simulink model "gm_sampleModel1590_sub"  (R2023a)
settings: Solver=VariableStepAuto  StartTime=0.0  StopTime=10.0  RelTol=1e-3
libraries: simulink x1, hdlsllib x1
settings Model: Creator=user1  LastModifiedBy=user1
settings OptimizationCC: BlockReduction=off  ConditionallyExecuteInputs=off
settings DebuggingCC: InheritedTsInSrcMsg=none

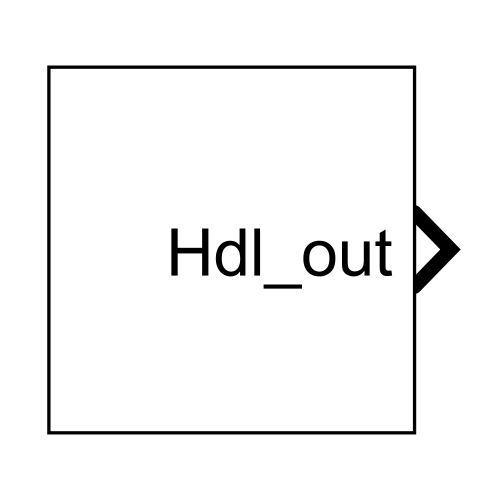
[thumbnail: Simulink's stored preview of the top-level diagram]
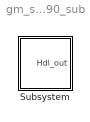
== system gm_sampleModel1590_sub ==
  Subsystem : Subsystem

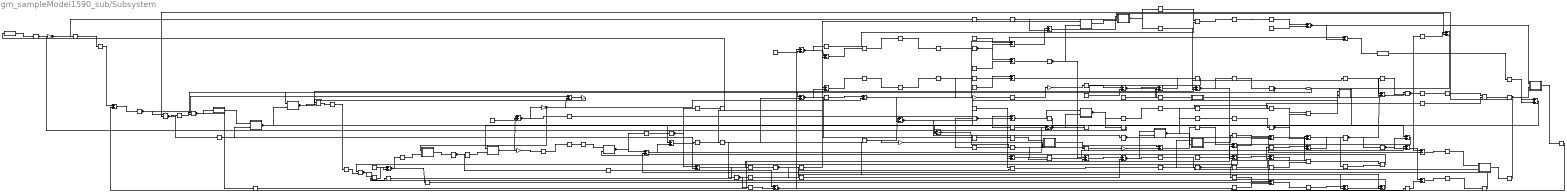
== system gm_sampleModel1590_sub/Subsystem ==
  Reshape{,1..6} (7 alike) : Reshape
  cfblk1 : Subsystem  mask(Detect Fall Nonpositive){vinit=double(0), InputProcessing=Elements as channels (sample based), OutDataTypeStr=uint8}
      mask prompts: vinit "Simulink:masks:InitialCondition_MP"; InputProcessing "Simulink:masks:InputProcessing_MP"; OutDataTypeStr "Simulink:masks:OutputDataType_MP"
      mask help: Simulink:masks:DetectFallNonpositive_MD
      mask init:
      | InputProcessing = 'Elements as channels (sample based)';
      | OutDataTypeStr = 'uint8';
      | vinit = double(0);
      mask TypeOptions InputProcessing: Simulink:masks:ColumnsAsChannelsFrameBased | Simulink:masks:ElementsAsChannelsSampleBased
      mask TypeOptions OutDataTypeStr: Simulink:masks:uint8 | Simulink:masks:boolean
      mask Display: fprintf('U <= 0\n&  NOT\nU/z <= 0')
  cfblk{10..11,18,20,23,31,51,76,82,92..93,104,106,117,120,125,127,131,137,139,145} (21 alike) : Signum  SampleTime=1
  cfblk{43,50,54,72,95,100,114,142} (8 alike) : Gain  Gain="fi(0,0,8,7,\"hex\",\"80\")"  ParamDataTypeStr=fixdt(0, 8, 7)  OutDataTypeStr=uint8  SampleTime=1
  cfblk{27,38,70..71,101,123,130,133,136,150} (10 alike) : Sum  Inputs=+  OutDataTypeStr=uint8
  cfblk102_inst : Subsystem
  cfblk{19,42,58,61,63,77,87,103,110,112,115,140} (12 alike) : Product  Inputs=*/  OutDataTypeStr=uint8  RndMeth=Zero  SaturateOnIntegerOverflow=on  SampleTime=1
  cfblk{4,33,45,60,74,84,89,105,121..122,134,147} (12 alike) : Sum  AccumDataTypeStr=uint8  OutDataTypeStr=uint8  RndMeth=Nearest  SampleTime=1
  cfblk105_const_val : Constant  Value=0  VectorParams1D=off  OutDataTypeStr=uint8  SampleTime=1
  cfblk{8,29,34,36,48..49,56..57,64,66,78,85..86,94,97,107,111,129,143..144} (20 alike) : Sum  AccumDataTypeStr=uint8  OutDataTypeStr=uint8  SampleTime=1
  cfblk{16,21,24,28,30,55,62,68,81,96,109,118} (12 alike) : Abs  SampleTime=1  OutDataTypeStr=uint8  SaturateOnIntegerOverflow=off
  cfblk{6,25..26,35,37,39..40,47,52..53,69,80,91,99,113,116,141,152} (18 alike) : MinMax  OutDataTypeStr=uint8
  cfblk{5,15,59,67,73,79,83,90,119,124,128,132} (12 alike) : Sum  Inputs=+-  AccumDataTypeStr=uint8  OutDataTypeStr=uint8  SampleTime=1
  cfblk121_const_val : Constant  Value=0  VectorParams1D=off  OutDataTypeStr=uint8  SampleTime=1
  cfblk122_const_val : Constant  Value=0  VectorParams1D=off  OutDataTypeStr=uint8  SampleTime=1
  cfblk126_inst : Subsystem
  cfblk134_const_val : Constant  Value=0  VectorParams1D=off  OutDataTypeStr=uint8  SampleTime=1
  cfblk135_inst : Subsystem
  cfblk13_inst : Subsystem
  cfblk146_inst : Subsystem
  cfblk147_const_val : Constant  Value=0  VectorParams1D=off  OutDataTypeStr=uint8  SampleTime=1
  cfblk148_inst : Subsystem
  cfblk149_inst : Subsystem
  cfblk158 : Constant  OutDataTypeStr=uint8  SampleTime=1
  cfblk159 : Constant  OutDataTypeStr=uint8  SampleTime=1
  cfblk160 : Constant  Value=0  VectorParams1D=off  OutDataTypeStr=uint8  SampleTime=1
  cfblk161 : Subsystem
  cfblk162 : Subsystem
  cfblk164 : Switch  Threshold=double(0)  OutDataTypeStr=uint8  SampleTime=1  SaturateOnIntegerOverflow=off  InputSameDT=off
  cfblk165 : Switch  Threshold=double(0)  OutDataTypeStr=uint8  SampleTime=1  SaturateOnIntegerOverflow=off  InputSameDT=off
  cfblk{166..190} (25 alike) : Delay  DelayLength=double(2)  InitialCondition=0  SampleTime=1
  cfblk17_inst : Subsystem
  cfblk{191..192,194..195} (4 alike) : DataTypeConversion  OutDataTypeStr=fixdt(0,8,0)
  cfblk193 : DataTypeConversion  OutDataTypeStr=uint8  SampleTime=1  SaturateOnIntegerOverflow=off  RndMeth=Floor
  cfblk2 : simulink/Logic and Bit Operations/Detect Increase  vinit=0.0  OutDataTypeStr=uint8
      settings: LibrarySourceBlock=|
      | hdlsllib/Logic and Bit
      | Operations/Detect
      | Increase
  cfblk3 : hdlsllib/Logic and Bit Operations/Bit Concat  numInputs=2
  cfblk32_inst : Subsystem
  cfblk33_const_val : Constant  Value=0  VectorParams1D=off  OutDataTypeStr=uint8  SampleTime=1
  cfblk44_inst : Subsystem
  cfblk45_const_val : Constant  Value=0  VectorParams1D=off  OutDataTypeStr=uint8  SampleTime=1
  cfblk4_const_val : Constant  Value=0  VectorParams1D=off  OutDataTypeStr=uint8  SampleTime=1
  cfblk60_const_val : Constant  Value=0  VectorParams1D=off  OutDataTypeStr=uint8  SampleTime=1
  cfblk65_inst : Subsystem
  cfblk74_const_val : Constant  Value=0  VectorParams1D=off  OutDataTypeStr=uint8  SampleTime=1
  cfblk84_const_val : Constant  Value=0  VectorParams1D=off  OutDataTypeStr=uint8  SampleTime=1
  cfblk88_inst : Subsystem
  cfblk89_const_val : Constant  Value=0  VectorParams1D=off  OutDataTypeStr=uint8  SampleTime=1
  cfblk98_inst : Subsystem
  cfblk9_inst : Subsystem
  Hdl_out : Outport  OutDataTypeStr=uint8  SampleTime=1
  wires:
  cfblk1/1(Y) -> cfblk191/1
  cfblk10/1 -> Reshape3/1
  cfblk100/1 -> cfblk97/2
  cfblk101/1 -> cfblk70/1
  cfblk102_inst/1(out1) -> cfblk176/1, cfblk80/1
  cfblk103/1 -> cfblk120/1, cfblk162/1(In1)
  cfblk104/1 -> cfblk146_inst/2(in2)
  cfblk105/1 -> cfblk63/1
  cfblk106/1 -> cfblk188/1
  cfblk107/1 -> cfblk48/2, cfblk20/1, cfblk145/1, cfblk13_inst/1(in1)
  Reshape/1 -> cfblk122/1
  cfblk109/1 -> cfblk126_inst/1(in1), cfblk119/2
  cfblk11/1 -> cfblk82/1
  cfblk110/1 -> cfblk123/1
  cfblk111/1 -> cfblk124/2, cfblk26/1
  cfblk112/1 -> cfblk84/1
  cfblk113/1 -> cfblk98_inst/1(in1)
  cfblk114/1 -> cfblk141/1
  cfblk115/1 -> cfblk146_inst/1(in1)
  cfblk116/1 -> cfblk57/2, cfblk115/2
  cfblk117/1 -> cfblk29/1, cfblk189/1
  cfblk118/1 -> cfblk90/2, cfblk137/1, cfblk107/2
  cfblk119/1 -> cfblk113/1
  Reshape1/1 -> cfblk194/1
  cfblk120/1 -> cfblk124/1
  cfblk121/1 -> cfblk185/1
  cfblk122/1 -> cfblk49/2
  cfblk123/1 -> cfblk98_inst/2(in2), cfblk149_inst/1(in1)
  cfblk124/1 -> cfblk105/1
  cfblk125/1 -> cfblk177/1
  cfblk126_inst/1(out1) -> cfblk149_inst/2(in2), cfblk10/1, cfblk186/1
  cfblk127/1 -> cfblk4/1
  cfblk128/1 -> cfblk16/1
  cfblk129/1 -> cfblk6/1
  cfblk13_inst/1(out1) -> cfblk65_inst/2(in2)
  cfblk130/1 -> cfblk101/1
  cfblk131/1 -> cfblk94/1
  cfblk132/1 -> cfblk2/1
  cfblk133/1 -> cfblk8/2, cfblk5/2
  cfblk134/1 -> cfblk104/1, cfblk54/1
  cfblk135_inst/1(out1) -> cfblk111/1, cfblk61/2
  cfblk136/1 -> cfblk106/1
  cfblk137/1 -> cfblk24/1, cfblk174/1
  cfblk139/1 -> cfblk8/1
  Reshape2/1 -> cfblk79/1
  cfblk140/1 -> cfblk139/1, Reshape1/1, cfblk119/1
  cfblk141/1 -> cfblk95/1
  cfblk142/1 -> cfblk136/1
  cfblk143/1 -> cfblk39/1
  cfblk144/1 -> cfblk77/1
  cfblk145/1 -> cfblk66/1
  cfblk146_inst/1(out1) -> cfblk129/1
  cfblk147/1 -> cfblk40/1
  cfblk148_inst/1(out1) -> cfblk85/2, cfblk135_inst/2(in2)
  cfblk149_inst/1(out1) -> cfblk172/1
  cfblk15/1 -> cfblk5/1
  cfblk150/1 -> cfblk56/2, cfblk144/2
  Reshape3/1 -> cfblk116/1
  cfblk152/1 -> cfblk167/1
  cfblk158/1 -> cfblk59/1, cfblk72/1
  cfblk159/1 -> cfblk15/1
  cfblk16/1 -> cfblk93/1
  cfblk160/1 -> cfblk63/2
  cfblk161/1(Out1) -> cfblk184/1
  cfblk162/1(Out1) -> cfblk148_inst/1(in1)
  cfblk164/1 -> cfblk18/1, cfblk102_inst/2(in2)
  cfblk165/1 -> cfblk81/1, cfblk38/1, cfblk52/1
  cfblk166/1 -> cfblk32_inst/2(in2)
  cfblk167/1 -> cfblk73/2
  cfblk168/1 -> cfblk79/2
  cfblk169/1 -> cfblk36/1
  cfblk17_inst/1(out1) -> cfblk92/1
  cfblk170/1 -> cfblk111/2
  cfblk171/1 -> cfblk58/2
  cfblk172/1 -> cfblk49/1
  cfblk173/1 -> cfblk19/2
  cfblk174/1 -> cfblk94/2
  cfblk175/1 -> cfblk17_inst/2(in2)
  cfblk176/1 -> cfblk164/1
  cfblk177/1 -> cfblk115/1
  cfblk178/1 -> cfblk165/2
  cfblk179/1 -> cfblk164/3
  cfblk18/1 -> cfblk165/1
  cfblk180/1 -> cfblk9_inst/1(in1)
  cfblk181/1 -> cfblk34/2
  cfblk182/1 -> cfblk128/2
  cfblk183/1 -> cfblk67/1
  cfblk184/1 -> cfblk140/2
  cfblk185/1 -> cfblk135_inst/1(in1)
  cfblk186/1 -> cfblk195/1
  cfblk187/1 -> cfblk143/1
  cfblk188/1 -> cfblk44_inst/1(in1)
  cfblk189/1 -> cfblk192/1
  cfblk19/1 -> Reshape4/1, cfblk47/1
  cfblk190/1 -> cfblk103/2, Hdl_out/1
  cfblk191/1 -> cfblk109/1, cfblk50/1
  cfblk192/1 -> cfblk1/1(U)
  cfblk193/1 -> cfblk88_inst/2(in2), cfblk36/2
  cfblk194/1 -> cfblk3/1
  cfblk195/1 -> cfblk3/2
  cfblk2/1 -> cfblk169/1
  cfblk20/1 -> cfblk164/2, cfblk42/1
  cfblk21/1 -> cfblk53/1
  cfblk23/1 -> cfblk21/1
  cfblk24/1 -> cfblk110/2
  cfblk25/1 -> cfblk78/1, cfblk19/1
  cfblk26/1 -> cfblk190/1
  cfblk27/1 -> cfblk83/2
  cfblk28/1 -> cfblk100/1
  cfblk29/1 -> cfblk86/2
  cfblk3/1 -> cfblk193/1
  cfblk30/1 -> cfblk56/1
  cfblk31/1 -> cfblk77/2
  cfblk32_inst/1(out1) -> cfblk134/1, cfblk142/1
  cfblk33/1 -> Reshape5/1
  cfblk34/1 -> cfblk55/1, cfblk126_inst/2(in2)
  cfblk35/1 -> cfblk87/1
  cfblk36/1 -> cfblk32_inst/1(in1)
  cfblk37/1 -> Reshape2/1
  cfblk38/1 -> cfblk85/1, cfblk45/1, cfblk179/1
  cfblk39/1 -> cfblk67/2, cfblk150/1
  cfblk4/1 -> cfblk62/1, cfblk121/1
  cfblk40/1 -> cfblk64/1
  Reshape4/1 -> cfblk103/1
  cfblk42/1 -> cfblk57/1
  cfblk43/1 -> cfblk61/1
  cfblk44_inst/1(out1) -> cfblk73/1, cfblk91/1
  cfblk45/1 -> cfblk102_inst/1(in1), cfblk178/1
  Reshape5/1 -> cfblk86/1, cfblk13_inst/2(in2)
  cfblk47/1 -> cfblk29/2, cfblk148_inst/2(in2)
  cfblk48/1 -> cfblk130/1
  cfblk49/1 -> cfblk143/2
  cfblk5/1 -> cfblk65_inst/1(in1)
  cfblk50/1 -> cfblk37/1, cfblk71/1
  cfblk51/1 -> cfblk76/1, cfblk187/1
  cfblk52/1 -> cfblk110/1
  cfblk53/1 -> cfblk64/2, cfblk182/1, cfblk181/1
  cfblk54/1 -> cfblk78/2, cfblk66/2, cfblk17_inst/1(in1)
  cfblk55/1 -> cfblk51/1
  cfblk56/1 -> cfblk83/1
  cfblk57/1 -> cfblk171/1
  cfblk58/1 -> cfblk44_inst/2(in2)
  cfblk59/1 -> cfblk165/3, cfblk144/1
  cfblk6/1 -> cfblk48/1, cfblk118/1
  cfblk60/1 -> cfblk88_inst/1(in1), cfblk132/2
  cfblk61/1 -> cfblk68/1
  cfblk62/1 -> cfblk161/1(In1)
  cfblk63/1 -> cfblk58/1
  cfblk64/1 -> cfblk90/1
  cfblk65_inst/1(out1) -> cfblk170/1, cfblk35/1
  cfblk66/1 -> cfblk59/2, cfblk132/1
  cfblk67/1 -> cfblk140/1
  cfblk68/1 -> cfblk31/1
  cfblk69/1 -> cfblk33/1, cfblk15/2
  cfblk70/1 -> Reshape6/1, cfblk114/1
  cfblk71/1 -> cfblk133/1
  cfblk72/1 -> cfblk97/1
  cfblk73/1 -> cfblk9_inst/2(in2), cfblk129/2
  cfblk74/1 -> cfblk183/1
  Reshape6/1 -> cfblk74/1
  cfblk76/1 -> cfblk147/1
  cfblk77/1 -> cfblk23/1, cfblk112/1
  cfblk78/1 -> cfblk43/1
  cfblk79/1 -> cfblk25/1
  cfblk8/1 -> cfblk107/1
  cfblk80/1 -> cfblk125/1
  cfblk81/1 -> cfblk180/1
  cfblk82/1 -> cfblk60/1
  cfblk83/1 -> cfblk152/1
  cfblk84/1 -> cfblk30/1, cfblk175/1
  cfblk85/1 -> cfblk42/2
  cfblk86/1 -> cfblk34/1
  cfblk87/1 -> cfblk11/1
  cfblk88_inst/1(out1) -> cfblk168/1
  cfblk89/1 -> cfblk128/1, cfblk99/1
  cfblk9_inst/1(out1) -> cfblk28/1
  cfblk90/1 -> cfblk112/2
  cfblk91/1 -> cfblk117/1
  cfblk92/1 -> cfblk131/1, cfblk166/1
  cfblk93/1 -> cfblk96/1
  cfblk94/1 -> cfblk89/1, cfblk27/1
  cfblk95/1 -> cfblk127/1
  cfblk96/1 -> cfblk69/1
  cfblk97/1 -> Reshape/1
  cfblk98_inst/1(out1) -> cfblk173/1
  cfblk99/1 -> cfblk87/2
  cfblk105_const_val/1 -> cfblk105/2
  cfblk121_const_val/1 -> cfblk121/2
  cfblk122_const_val/1 -> cfblk122/2
  cfblk134_const_val/1 -> cfblk134/2
  cfblk147_const_val/1 -> cfblk147/2
  cfblk33_const_val/1 -> cfblk33/2
  cfblk4_const_val/1 -> cfblk4/2
  cfblk45_const_val/1 -> cfblk45/2
  cfblk60_const_val/1 -> cfblk60/2
  cfblk74_const_val/1 -> cfblk74/2
  cfblk84_const_val/1 -> cfblk84/2
  cfblk89_const_val/1 -> cfblk89/2

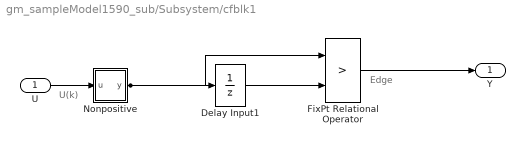
== system gm_sampleModel1590_sub/Subsystem/cfblk1 ==
  note: U(k)
  note: Edge
  U : Inport  OutDataTypeStr=uint8  SampleTime=1
  Delay Input1 : UnitDelay  Description=Store in Global RAM  DisableCoverage=on  InitialCondition=vinit  SampleTime=-1  HasFrameUpgradeWarning=on
  FixPt Relational Operator : RelationalOperator  Operator=>  OutDataTypeStr=fixdt(0, 8)  ZeroCross=off  InputSameDT=off
  Nonpositive : Subsystem  mask(Compare To Zero){relop=<=, OutDataTypeStr=boolean, ZeroCross=off}
      mask prompts: relop "Simulink:masks:Operator_MP"; OutDataTypeStr "Simulink:masks:OutputDataType_MP"; ZeroCross "Simulink:masks:EnableZerocrossingDetection_MP"
      mask help: Simulink:masks:CompareToZero_MD
      mask init:
      | OutDataTypeStr = 'boolean';
      | ZeroCross = 'off';
      | blkName = 'sampleModel1590_sub/Subsystem/cfblk1/Nonpositive';
      | relop = '<=';
      | setValue = 'boolean';
      mask TypeOptions relop: == | ~= | < | <= | >= | >
      mask TypeOptions OutDataTypeStr: Simulink:masks:uint8 | Simulink:masks:boolean
      mask Callback ZeroCross: sl('zeroCrossEnable', gcbh);
      mask Display: disp([relop,' 0'])
  Y : Outport  SampleTime=1
  wires:
  U/1 -> Nonpositive/1(u)
  Delay Input1/1 -> FixPt Relational Operator/2
  FixPt Relational Operator/1 -> Y/1
  Nonpositive/1(y) -> FixPt Relational Operator/1, Delay Input1/1

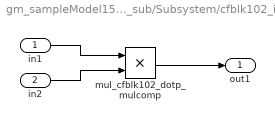
== system gm_sampleModel1590_sub/Subsystem/cfblk102_inst ==
  in1 : Inport  OutDataTypeStr=uint8  SampleTime=1
  in2 : Inport  Port=2  OutDataTypeStr=uint8  SampleTime=1
  mul_cfblk102_dotp_mulcomp : Product  Inputs=**  OutDataTypeStr=uint8  SampleTime=1
  out1 : Outport  OutDataTypeStr=uint8  SampleTime=1
  wires:
  in1/1 -> mul_cfblk102_dotp_mulcomp/1
  in2/1 -> mul_cfblk102_dotp_mulcomp/2
  mul_cfblk102_dotp_mulcomp/1 -> out1/1

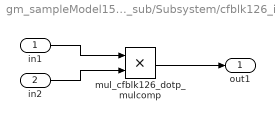
== system gm_sampleModel1590_sub/Subsystem/cfblk126_inst ==
  in1 : Inport  OutDataTypeStr=uint8  SampleTime=1
  in2 : Inport  Port=2  OutDataTypeStr=uint8  SampleTime=1
  mul_cfblk126_dotp_mulcomp : Product  Inputs=**  OutDataTypeStr=uint8  SampleTime=1
  out1 : Outport  OutDataTypeStr=uint8  SampleTime=1
  wires:
  in1/1 -> mul_cfblk126_dotp_mulcomp/1
  in2/1 -> mul_cfblk126_dotp_mulcomp/2
  mul_cfblk126_dotp_mulcomp/1 -> out1/1

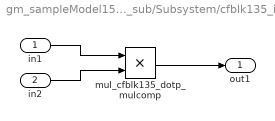
== system gm_sampleModel1590_sub/Subsystem/cfblk135_inst ==
  in1 : Inport  OutDataTypeStr=uint8  SampleTime=1
  in2 : Inport  Port=2  OutDataTypeStr=uint8  SampleTime=1
  mul_cfblk135_dotp_mulcomp : Product  Inputs=**  OutDataTypeStr=uint8  SampleTime=1
  out1 : Outport  OutDataTypeStr=uint8  SampleTime=1
  wires:
  in1/1 -> mul_cfblk135_dotp_mulcomp/1
  in2/1 -> mul_cfblk135_dotp_mulcomp/2
  mul_cfblk135_dotp_mulcomp/1 -> out1/1

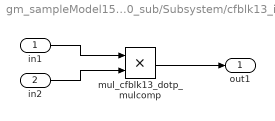
== system gm_sampleModel1590_sub/Subsystem/cfblk13_inst ==
  in1 : Inport  OutDataTypeStr=uint8  SampleTime=1
  in2 : Inport  Port=2  OutDataTypeStr=uint8  SampleTime=1
  mul_cfblk13_dotp_mulcomp : Product  Inputs=**  OutDataTypeStr=uint8  SampleTime=1
  out1 : Outport  OutDataTypeStr=uint8  SampleTime=1
  wires:
  in1/1 -> mul_cfblk13_dotp_mulcomp/1
  in2/1 -> mul_cfblk13_dotp_mulcomp/2
  mul_cfblk13_dotp_mulcomp/1 -> out1/1

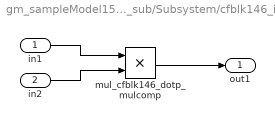
== system gm_sampleModel1590_sub/Subsystem/cfblk146_inst ==
  in1 : Inport  OutDataTypeStr=uint8  SampleTime=1
  in2 : Inport  Port=2  OutDataTypeStr=uint8  SampleTime=1
  mul_cfblk146_dotp_mulcomp : Product  Inputs=**  OutDataTypeStr=uint8  SampleTime=1
  out1 : Outport  OutDataTypeStr=uint8  SampleTime=1
  wires:
  in1/1 -> mul_cfblk146_dotp_mulcomp/1
  in2/1 -> mul_cfblk146_dotp_mulcomp/2
  mul_cfblk146_dotp_mulcomp/1 -> out1/1

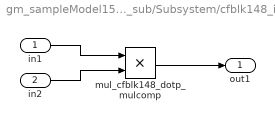
== system gm_sampleModel1590_sub/Subsystem/cfblk148_inst ==
  in1 : Inport  OutDataTypeStr=uint8  SampleTime=1
  in2 : Inport  Port=2  OutDataTypeStr=uint8  SampleTime=1
  mul_cfblk148_dotp_mulcomp : Product  Inputs=**  OutDataTypeStr=uint8  SampleTime=1
  out1 : Outport  OutDataTypeStr=uint8  SampleTime=1
  wires:
  in1/1 -> mul_cfblk148_dotp_mulcomp/1
  in2/1 -> mul_cfblk148_dotp_mulcomp/2
  mul_cfblk148_dotp_mulcomp/1 -> out1/1

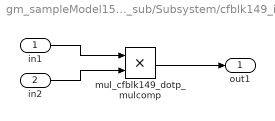
== system gm_sampleModel1590_sub/Subsystem/cfblk149_inst ==
  in1 : Inport  OutDataTypeStr=uint8  SampleTime=1
  in2 : Inport  Port=2  OutDataTypeStr=uint8  SampleTime=1
  mul_cfblk149_dotp_mulcomp : Product  Inputs=**  OutDataTypeStr=uint8  SampleTime=1
  out1 : Outport  OutDataTypeStr=uint8  SampleTime=1
  wires:
  in1/1 -> mul_cfblk149_dotp_mulcomp/1
  in2/1 -> mul_cfblk149_dotp_mulcomp/2
  mul_cfblk149_dotp_mulcomp/1 -> out1/1

== system gm_sampleModel1590_sub/Subsystem/cfblk161 ==
  In1 : Inport  OutDataTypeStr=uint8  PortDimensions=1  SampleTime=1
  Out1 : Outport  SampleTime=1
  wires:
  In1/1 -> Out1/1

== system gm_sampleModel1590_sub/Subsystem/cfblk162 ==
  In1 : Inport  OutDataTypeStr=uint8  PortDimensions=1  SampleTime=1
  Out1 : Outport  SampleTime=1
  wires:
  In1/1 -> Out1/1

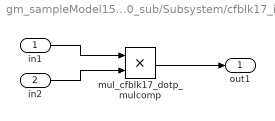
== system gm_sampleModel1590_sub/Subsystem/cfblk17_inst ==
  in1 : Inport  OutDataTypeStr=uint8  SampleTime=1
  in2 : Inport  Port=2  OutDataTypeStr=uint8  SampleTime=1
  mul_cfblk17_dotp_mulcomp : Product  Inputs=**  OutDataTypeStr=uint8  SampleTime=1
  out1 : Outport  OutDataTypeStr=uint8  SampleTime=1
  wires:
  in1/1 -> mul_cfblk17_dotp_mulcomp/1
  in2/1 -> mul_cfblk17_dotp_mulcomp/2
  mul_cfblk17_dotp_mulcomp/1 -> out1/1

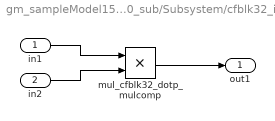
== system gm_sampleModel1590_sub/Subsystem/cfblk32_inst ==
  in1 : Inport  OutDataTypeStr=uint8  SampleTime=1
  in2 : Inport  Port=2  OutDataTypeStr=uint8  SampleTime=1
  mul_cfblk32_dotp_mulcomp : Product  Inputs=**  OutDataTypeStr=uint8  SampleTime=1
  out1 : Outport  OutDataTypeStr=uint8  SampleTime=1
  wires:
  in1/1 -> mul_cfblk32_dotp_mulcomp/1
  in2/1 -> mul_cfblk32_dotp_mulcomp/2
  mul_cfblk32_dotp_mulcomp/1 -> out1/1

== system gm_sampleModel1590_sub/Subsystem/cfblk44_inst ==
  in1 : Inport  OutDataTypeStr=uint8  SampleTime=1
  in2 : Inport  Port=2  OutDataTypeStr=uint8  SampleTime=1
  mul_cfblk44_dotp_mulcomp : Product  Inputs=**  OutDataTypeStr=uint8  SampleTime=1
  out1 : Outport  OutDataTypeStr=uint8  SampleTime=1
  wires:
  in1/1 -> mul_cfblk44_dotp_mulcomp/1
  in2/1 -> mul_cfblk44_dotp_mulcomp/2
  mul_cfblk44_dotp_mulcomp/1 -> out1/1

== system gm_sampleModel1590_sub/Subsystem/cfblk65_inst ==
  in1 : Inport  OutDataTypeStr=uint8  SampleTime=1
  in2 : Inport  Port=2  OutDataTypeStr=uint8  SampleTime=1
  mul_cfblk65_dotp_mulcomp : Product  Inputs=**  OutDataTypeStr=uint8  SampleTime=1
  out1 : Outport  OutDataTypeStr=uint8  SampleTime=1
  wires:
  in1/1 -> mul_cfblk65_dotp_mulcomp/1
  in2/1 -> mul_cfblk65_dotp_mulcomp/2
  mul_cfblk65_dotp_mulcomp/1 -> out1/1

== system gm_sampleModel1590_sub/Subsystem/cfblk88_inst ==
  in1 : Inport  OutDataTypeStr=uint8  SampleTime=1
  in2 : Inport  Port=2  OutDataTypeStr=uint8  SampleTime=1
  mul_cfblk88_dotp_mulcomp : Product  Inputs=**  OutDataTypeStr=uint8  SampleTime=1
  out1 : Outport  OutDataTypeStr=uint8  SampleTime=1
  wires:
  in1/1 -> mul_cfblk88_dotp_mulcomp/1
  in2/1 -> mul_cfblk88_dotp_mulcomp/2
  mul_cfblk88_dotp_mulcomp/1 -> out1/1

== system gm_sampleModel1590_sub/Subsystem/cfblk98_inst ==
  in1 : Inport  OutDataTypeStr=uint8  SampleTime=1
  in2 : Inport  Port=2  OutDataTypeStr=uint8  SampleTime=1
  mul_cfblk98_dotp_mulcomp : Product  Inputs=**  OutDataTypeStr=uint8  SampleTime=1
  out1 : Outport  OutDataTypeStr=uint8  SampleTime=1
  wires:
  in1/1 -> mul_cfblk98_dotp_mulcomp/1
  in2/1 -> mul_cfblk98_dotp_mulcomp/2
  mul_cfblk98_dotp_mulcomp/1 -> out1/1

== system gm_sampleModel1590_sub/Subsystem/cfblk9_inst ==
  in1 : Inport  OutDataTypeStr=uint8  SampleTime=1
  in2 : Inport  Port=2  OutDataTypeStr=uint8  SampleTime=1
  mul_cfblk9_dotp_mulcomp : Product  Inputs=**  OutDataTypeStr=uint8  SampleTime=1
  out1 : Outport  OutDataTypeStr=uint8  SampleTime=1
  wires:
  in1/1 -> mul_cfblk9_dotp_mulcomp/1
  in2/1 -> mul_cfblk9_dotp_mulcomp/2
  mul_cfblk9_dotp_mulcomp/1 -> out1/1

== system gm_sampleModel1590_sub/Subsystem/cfblk1/Nonpositive ==
  u : Inport  OutDataTypeStr=uint8  SampleTime=1
  Compare : RelationalOperator  Operator=<=  OutDataTypeStr=boolean  ZeroCross=off
  Constant : Constant  DisableCoverage=on  Value=0  OutDataTypeStr=Inherit: Inherit via back propagation  SampleTime=-1  PreserveConstantTs=on
  y : Outport  SampleTime=1
  wires:
  u/1 -> Compare/1
  Compare/1 -> y/1
  Constant/1 -> Compare/2
